simulink model "Experiment1_optional_simulink"  (R2024b)
settings: Solver=VariableStepAuto  StartTime=0.0  StopTime=1  RelTol=1e-3
values from neighbouring files (symbols this model uses):
  d = 0.165    [EX_opt_1.m]
  r = 0.03    [EX_opt_1.m]
  theta_0 = 0    [EX_opt_1.m]
  v_d = 0    [EX_opt_1.m]
  w_d = 2    [EX_opt_1.m]
  x_0 = 1    [EX_opt_1.m]
  y_0 = 1    [EX_opt_1.m]
settings Model: Creator=sofiagirardello  LastModifiedBy=leontecosm
settings RTWCC: GPUComputeCapability=3.5

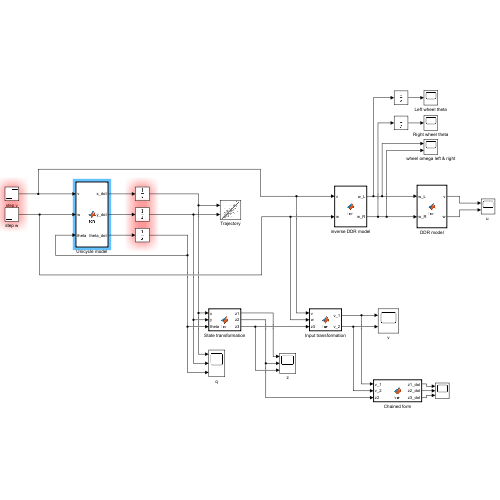
[thumbnail: Simulink's stored preview of the top-level diagram]
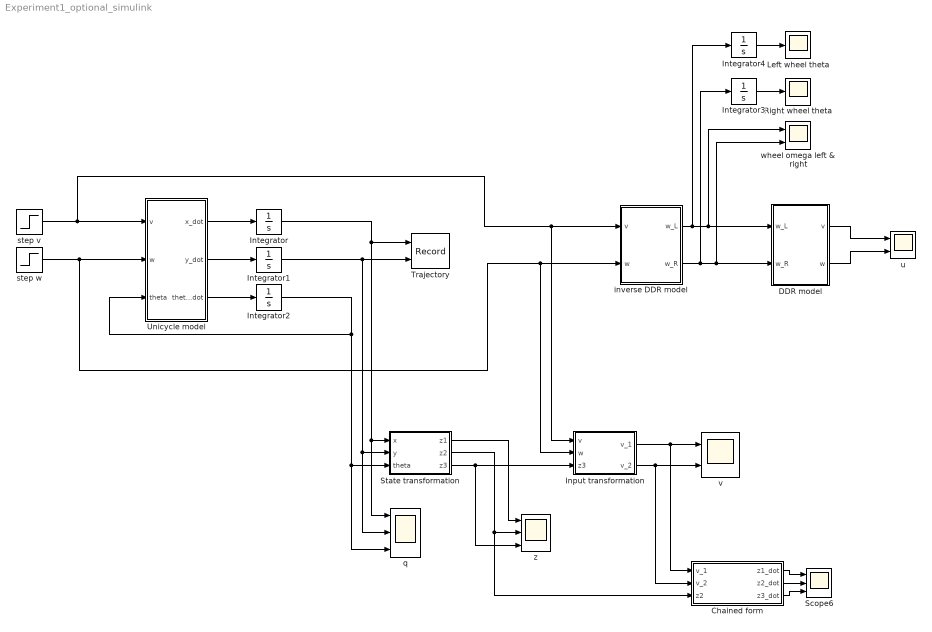
== system Experiment1_optional_simulink ==
  Chained form : MATLAB Function  TreatAsAtomicUnit=on
  DDR model : MATLAB Function  TreatAsAtomicUnit=on
  Input transformation : MATLAB Function  TreatAsAtomicUnit=on
  Integrator : Integrator  InitialCondition=x_0
  Integrator1 : Integrator  InitialCondition=y_0
  Integrator2 : Integrator  InitialCondition=theta_0
  Integrator3 : Integrator
  Integrator4 : Integrator
  Left wheel theta : Scope
  Right wheel theta : Scope
  Scope6 : Scope  NumInputPorts=3
  State transformation : MATLAB Function  TreatAsAtomicUnit=on
  Trajectory : Record  FileSettingsInternal="{\"entries\":[{\"content\":{\"excelSettings\":{\"content\":{},\"type\":\"Streamout.ExcelSettings\"}},\"type\":\"Streamout.FileSettingStorage\",\"uuid\":\"\"}],\"packageUris\":[\"http:\\/\\/schema.mathworks.com\\/mf0\\/streamout_blocks\\/R2020a\"],\"version\":\"1.0\"}"  Layout=[1 1]  SignalsInternal="{\"entries\":[{\"content\":{\"signals\":[{\"content\":{\"blockPath\":[],\"dimensions\":[1],\"domain\":\"\",\"lineColor\":\"#a2142f\",\"plots\":[ 1 ],\"port\":1,\"signalID\":1,\"signalName\":\"Integrator\"},\"type\":\"RecordBlkView.Signal\",\"uuid\":\"\"},{\"content\":{\"blockPath\":[],\"dimensions\":[1],\"domain\":\"\",\"lineColor\":\"#139fff\",\"plots\":[ 1 ],\"port\":2,\"signalID\":2,\"signalName\":\"Integrator1\"},\"type\":\"RecordBlkView.Signal\",\"uuid\":\"\"}]},\"type\":\"RecordBlkView.InputSignals\",\"uuid\":\"\"}],\"packageUris\":[\"http:\\/\\/schema.mathworks.com\\/mf0\\/streamout_blocks\\/R2020a\"],\"version\":\"1.0\"}"  VisualizationBindings="{\"xyplotplugin\":{\"info\":[{\"series\":[{\"bindingParametersList\":[{\"parameter\":\"X-Axis\",\"signalID\":1,\"signalName\":\"Integrator\"},{\"parameter\":\"Y-Axis\",\"signalID\":2,\"signalName\":\"Integrator1\"}],\"seriesID\":0}],\"subplotID\":1}]}}"  CompatibilityTag=XY
  Unicycle model : MATLAB Function  TreatAsAtomicUnit=on
  inverse DDR model : MATLAB Function  TreatAsAtomicUnit=on
  q : Scope  NumInputPorts=3
  step v : Step  Time=0  After=v_d  SampleTime=0
  step w : Step  Time=0  After=w_d  SampleTime=0
  "u " : Scope  NumInputPorts=2
  v : Scope  NumInputPorts=2
  wheel omega left & right : Scope  NumInputPorts=2
  z : Scope  NumInputPorts=3
  wires:
  Unicycle model/3(theta_dot) -> Integrator2/1
  inverse DDR model/2(w_R) -> Integrator3/1, wheel omega left & right/2, DDR model/2(w_R)
  Integrator1/1 -> q/2, State transformation/2(y), Trajectory/2
  Integrator2/1 -> State transformation/3(theta), q/3, Unicycle model/3(theta)
  Integrator3/1 -> Right wheel theta/1
  step w/1 -> Input transformation/2(w), inverse DDR model/2(w), Unicycle model/2(w)
  step v/1 -> Input transformation/1(v), inverse DDR model/1(v), Unicycle model/1(v)
  Unicycle model/2(y_dot) -> Integrator1/1
  Unicycle model/1(x_dot) -> Integrator/1
  Integrator/1 -> q/1, State transformation/1(x), Trajectory/1
  inverse DDR model/1(w_L) -> Integrator4/1, wheel omega left & right/1, DDR model/1(w_L)
  Integrator4/1 -> Left wheel theta/1
  State transformation/3(z3) -> z/3, Input transformation/3(z3)
  Input transformation/1(v_1) -> Chained form/1(v_1), v/1
  Input transformation/2(v_2) -> Chained form/2(v_2), v/2
  State transformation/2(z2) -> z/2, Chained form/3(z2)
  Chained form/1(z1_dot) -> Scope6/1
  Chained form/2(z2_dot) -> Scope6/2
  Chained form/3(z3_dot) -> Scope6/3
  DDR model/1(v) -> "u "/1
  DDR model/2(w) -> "u "/2
  State transformation/1(z1) -> z/1

== matlab function Experiment1_optional_simulink/Unicycle model ==
  data: v input; x_dot output; w input; theta input; y_dot output; theta_dot output
function  [x_dot, y_dot, theta_dot] = fcn(v,w,theta)
    
    x_dot = cos(theta)*v;
    y_dot = sin(theta)*v;
    theta_dot = w;

== matlab function Experiment1_optional_simulink/DDR model ==
  data: w_L input; v output; w output; w_R input; r parameter; d parameter
function [v,w] = fcn(w_L, w_R, r, d)

    v = (r/2)*w_L + (r/2)*w_R;
    w = -(r/d)*w_L +(r/d)*w_R;

== matlab function Experiment1_optional_simulink/inverse DDR model ==
  data: v input; w_L output; w input; w_R output; r parameter; d parameter
function [w_L,w_R]= fcn(v,w,r, d)

w_L = v/r - d*w/(2*r);
w_R = v/r + d*w/(2*r);

== matlab function Experiment1_optional_simulink/State transformation ==
  data: x input; z1 output; y input; theta input; z2 output; z3 output
function [z1, z2, z3] = fcn(x, y, theta)

z1 = theta;
z2 = cos(theta)*x + sin(theta)*y;
z3 = sin(theta)*x - cos(theta)*y;

== matlab function Experiment1_optional_simulink/Input transformation ==
  data: v input; v_1 output; w input; z3 input; v_2 output
function [v_1, v_2]= fcn(v,w,z3)

v_1 = w;
v_2 = v - z3*w;

== matlab function Experiment1_optional_simulink/Chained form ==
  data: v_1 input; z1_dot output; v_2 input; z2 input; z2_dot output; z3_dot output
function [z1_dot, z2_dot, z3_dot] = fcn(v_1,v_2,z2)

z1_dot = v_1;
z2_dot = v_2;
z3_dot = z2*v_1;
